simulink model "h175_model_cathode_harness_hctrl_basic"  (R2023a)
settings: Solver=VariableStepAuto  StartTime=0.0  StopTime=4750  RelTol=1e-2
InitFcn:
  | run("cathode_subsystem_parameters.m")
undefined symbols (not defined in the file or in its folder): sigbuilder_block
libraries: nesl_utility x12, fl_lib x10, simulink x5, slpidlib x2, eeGeneralControl x2, VariableTimeLowPassFilter x1
(part 2 of 2)

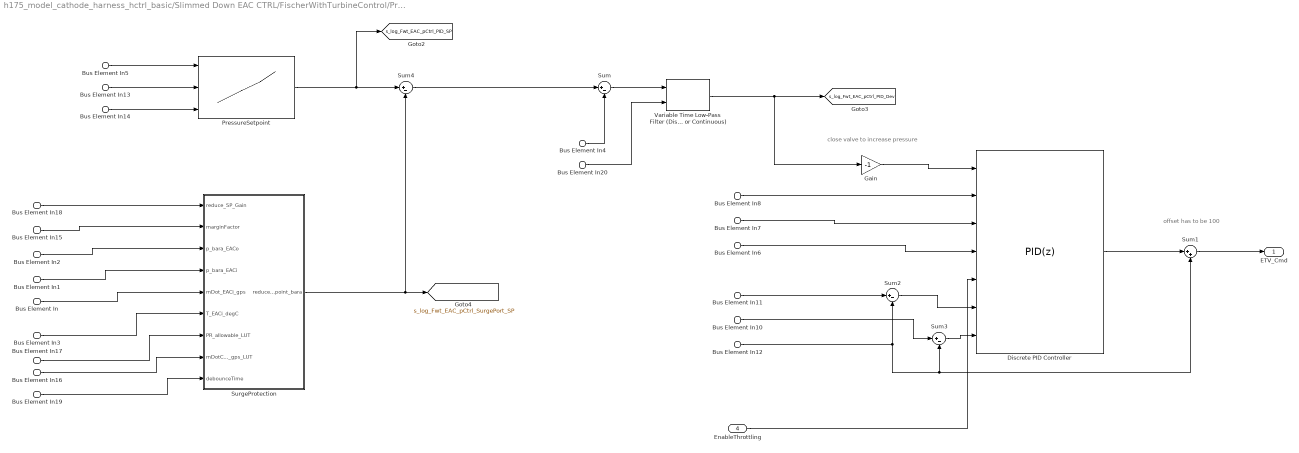
== system h175_model_cathode_harness_hctrl_basic/Slimmed Down EAC CTRL/FischerWithTurbineControl/PressureControl/AlternativeCathodePressureControl ==
  note: close valve to increase pressure
  note: offset has to be 100
  Bus Element In : Inport  PortName=CAT_Sensors  Element=b_mdotSens_EACi.s_mDot_gps_EACi_Get
  Bus Element In1 : Inport  PortName=CAT_Sensors  Element=b_pSens_EACi.s_p_bara_EACi_Get
  Bus Element In2 : Inport  PortName=CAT_Sensors  Element=b_pSens_EACo.s_p_bara_EACo_Get
  Bus Element In3 : Inport  PortName=CAT_Sensors  Element=b_TSens_EACi.s_T_degC_EACi_Get
  Bus Element In4 : Inport  PortName=CAT_Sensors  Element=b_pSens_CSti.s_p_bara_CSti_Get
  Bus Element In5 : Inport  Port=2  PortName=E_Sensors  Element=b_Sens_IVT.s_I_A_StN_Get
  Bus Element In6 : Inport  Port=3  PortName=EAC_Parameters  Element=p_Fwt_EAC_pCtrl_PID_D
  Bus Element In7 : Inport  Port=3  PortName=EAC_Parameters  Element=p_Fwt_EAC_pCtrl_PID_I
  Bus Element In8 : Inport  Port=3  PortName=EAC_Parameters  Element=p_Fwt_EAC_pCtrl_PID_P
  Bus Element In10 : Inport  Port=3  PortName=EAC_Parameters  Element=p_Fwt_EAC_pCtrl_PID_LowerLim_pos_per
  Bus Element In11 : Inport  Port=3  PortName=EAC_Parameters  Element=p_Fwt_EAC_pCtrl_PID_UpperLim_pos_per
  Bus Element In12 : Inport  Port=3  PortName=EAC_Parameters  Element=p_Fwt_EAC_pCtrl_PID_Offset_pos_per
  Bus Element In13 : Inport  Port=3  PortName=EAC_Parameters  Element=p_Fwt_EAC_pCtrl_SP_LUT_p_bara
  Bus Element In14 : Inport  Port=3  PortName=EAC_Parameters  Element=p_EAC_pCtrl_SP_LUT_I_A
  Bus Element In20 : Inport  Port=3  PortName=EAC_Parameters  Element=p_Fwt_EAC_pCtrl_PID_Filtr_T
  Bus Element In16 : Inport  Port=3  PortName=EAC_Parameters  Element=p_Fwt_EAC_pCtrl_SurgeProt_LUT_mDotCorr_gps
  Bus Element In17 : Inport  Port=3  PortName=EAC_Parameters  Element=p_Fwt_EAC_pCtrl_SurgeProt_LUT_PR
  Bus Element In15 : Inport  Port=3  PortName=EAC_Parameters  Element=p_Fwt_EAC_pCtrl_SurgeProt_PR_marginFactor
  Bus Element In18 : Inport  Port=3  PortName=EAC_Parameters  Element=p_Fwt_EAC_pCtrl_SurgeProt_redSP_Gain
  Bus Element In19 : Inport  Port=3  PortName=EAC_Parameters  Element=p_Fwt_EAC_pCtrl_SurgeProt_debounce_s
  EnableThrottling : Inport  Port=4
  Discrete PID Controller : slpidlib/PID Controller  Controller=PID  Form=Parallel  TimeDomain=Discrete-time  UseExternalTs=off  SampleTime=-1  IntegratorMethod=Trapezoidal  FilterMethod=Trapezoidal  ControllerParametersSource=external  P=1  I=1  UseKiTs=off  D=0  N=100  UseFilter=off  TunerSelectOption=Transfer Function Based (PID Tuner App)  InitialConditionSource=internal  InitialConditionForIntegrator=0  InitialConditionForFilter=0  DifferentiatorICPrevScaledInput=0  ExternalReset=either  TrackingMode=off  Kt=1  LimitOutput=on  SatLimitsSource=external  UpperSaturationLimit=inf  LowerSaturationLimit=-inf  LinearizeAsGain=off  AntiWindupMode=clamping  Kb=1  LimitIntegrator=off  UpperIntegratorSaturationLimit=inf  LowerIntegratorSaturationLimit=-inf  POutMin=[]  POutMax=[]  IOutMin=[]  IOutMax=[]  DOutMin=[]  DOutMax=[]  NOutMin=[]  NOutMax=[]  SumOutMin=[]  SumOutMax=[]  SaturationOutMin=[]  SaturationOutMax=[]  PParamMin=[]  PParamMax=[]  IParamMin=[]  IParamMax=[]  DParamMin=[]  DParamMax=[]  NParamMin=[]  NParamMax=[]  KbParamMin=[]  KbParamMax=[]  KtParamMin=[]  KtParamMax=[]  KbOutMin=[]  KbOutMax=[]  KtOutMin=[]  KtOutMax=[]  IntegratorOutMin=[]  IntegratorOutMax=[]  FilterOutMin=[]  FilterOutMax=[]  SumI1OutMin=[]  SumI1OutMax=[]  SumI2OutMin=[]  SumI2OutMax=[]  SumI3OutMin=[]  SumI3OutMax=[]  SumI4OutMin=[]  SumI4OutMax=[]  SumDOutMin=[]  SumDOutMax=[]  DifferentiatorOutMin=[]  DifferentiatorOutMax=[]  FilterDiffOutCoefMin=[]  FilterDiffOutCoefMax=[]  ReciprocalOutMin=[]  ReciprocalOutMax=[]  SumDenOutMin=[]  SumDenOutMax=[]  SumNumOutMin=[]  SumNumOutMax=[]  DivideOutMin=[]  DivideOutMax=[]  UdiffTsProdOutMin=[]  UdiffTsProdOutMax=[]  NTsProdOutMin=[]  NTsProdOutMax=[]  UintegralTsProdOutMin=[]  UintegralTsProdOutMax=[]  UngainTsProdOutMin=[]  UngainTsProdOutMax=[]  ClampingZeroOutDataTypeStr=Inherit: Inherit via back propagation  ClampingZeroOutMin=[]  ClampingZeroOutMax=[]  FilterDenConstantOutDataTypeStr=Inherit: Inherit via back propagation  FilterDenConstantOutMin=[]  FilterDenConstantOutMax=[]  PCopyOutDataTypeStr=Inherit: Inherit via back propagation  PCopyOutMin=[]  PCopyOutMax=[]  NCopyOutDataTypeStr=Inherit: Inherit via back propagation  NCopyOutMin=[]  NCopyOutMax=[]  IntegratorContinuousStateAttributes=''  IntegratorStateMustResolveToSignalObject=off  IntegratorRTWStateStorageClass=Auto  FilterContinuousStateAttributes=''  FilterStateMustResolveToSignalObject=off  FilterRTWStateStorageClass=Auto  ParallelPVariant=ExternalParameters  IdealPVariant=Disabled  IVariant=ExternalParameters  DVariant=ExternalParameters  IntegratorVariant=Discrete  SatVariant=External  AWVariant=DiscClampingParallel  PCopyVariant=Disabled  TRVariant=Disabled  FdbkBlocksVariant=Feedback  IdealPFdbkVariant=Passthrough  SatFdbkVariant=Passthrough  DerivativeFilterVariant=Differentiator  NVariant=Passthrough  NCopyVariant=Disabled_SignalSpec  FilterICVariant=InternalICsDifferentiator  IntegratorICVariant=InternalICs  ExternalResetVariant=ExternalReset  TRSumVariant=Passthrough  SumFdbkVariant=Enabled  SumVariant=Sum_PID  TsampFilterVariant=InternalTs  TsampNgainVariant=Passthrough  TsampIntegralVariant=Disabled_SignalSpec  ExternalSaturationOutDataTypeStr=Inherit: Same as second input
      settings: LibrarySourceBlock=simulink/Discrete/Discrete PID Controller
  Gain : Gain  Gain=-1
  PressureSetpoint : Lookup_n-D  NumberOfTableDimensions=1  BreakpointsForDimension1Source=Input port  BreakpointsForDimension1=[-5:5]  TableSource=Input port  Table=tanh([-5:5])  ExtrapMethod=Clip  InternalRulePriority=Speed  RndMeth=Simplest
      settings: InputPortMap=u0,p221,p5
  Sum{,2..4} (4 alike) : Sum  Inputs=|+-
  Sum1 : Sum  Inputs=|++
  SurgeProtection : Subsystem
  Variable Time Low-Pass Filter (Discrete or Continuous) : VariableTimeLowPassFilter/Variable Time Low-Pass Filter (Discrete or Continuous)  K=1  T=1  B=inf  A=-inf  init_option=Inherited from block input  x0=0  Ts=-1
      settings: LibrarySourceBlock=|
      | ee_sl_lib/General Control/Low-Pass Filter
      | (Discrete or Continuous)
  ETV_Cmd : Outport
  tag scope: s_log_Fwt_EAC_pCtrl_PID_Devi=global, s_log_Fwt_EAC_pCtrl_PID_SP=global, s_log_Fwt_EAC_pCtrl_SurgePort_SP=global
  wires:
  SurgeProtection/1(reducePressureSetpoint_bara) -> [s_log_Fwt_EAC_pCtrl_SurgePort_SP], Sum4/2
  Bus Element In19/1 -> SurgeProtection/9(debounceTime)
  Bus Element In16/1 -> SurgeProtection/8(mDotCorr_gps_LUT)
  Bus Element In17/1 -> SurgeProtection/7(PR_allowable_LUT)
  Bus Element In3/1 -> SurgeProtection/6(T_EACi_degC)
  Bus Element In/1 -> SurgeProtection/5(mDot_EACi_gps)
  Bus Element In1/1 -> SurgeProtection/4(p_bara_EACi)
  Bus Element In2/1 -> SurgeProtection/3(p_bara_EACo)
  Bus Element In15/1 -> SurgeProtection/2(marginFactor)
  Bus Element In18/1 -> SurgeProtection/1(reduce_SP_Gain)
  Bus Element In20/1 -> Variable Time Low-Pass Filter (Discrete or Continuous)/2
  Variable Time Low-Pass Filter (Discrete or Continuous)/1 -> [s_log_Fwt_EAC_pCtrl_PID_Devi], Gain/1
  Sum4/1 -> Sum/1
  PressureSetpoint/1 -> [s_log_Fwt_EAC_pCtrl_PID_SP], Sum4/1
  Bus Element In13/1 -> PressureSetpoint/2
  Bus Element In14/1 -> PressureSetpoint/3
  Discrete PID Controller/1 -> Sum1/1
  EnableThrottling/1 -> Discrete PID Controller/5
  Bus Element In7/1 -> Discrete PID Controller/3
  Sum/1 -> Variable Time Low-Pass Filter (Discrete or Continuous)/1
  Bus Element In8/1 -> Discrete PID Controller/2
  Sum3/1 -> Discrete PID Controller/7
  Bus Element In6/1 -> Discrete PID Controller/4
  Bus Element In11/1 -> Sum2/1
  Bus Element In12/1 -> Sum2/2, Sum3/2, Sum1/2
  Sum1/1 -> ETV_Cmd/1
  Sum2/1 -> Discrete PID Controller/6
  Bus Element In10/1 -> Sum3/1
  Gain/1 -> Discrete PID Controller/1
  Bus Element In5/1 -> PressureSetpoint/1
  Bus Element In4/1 -> Sum/2

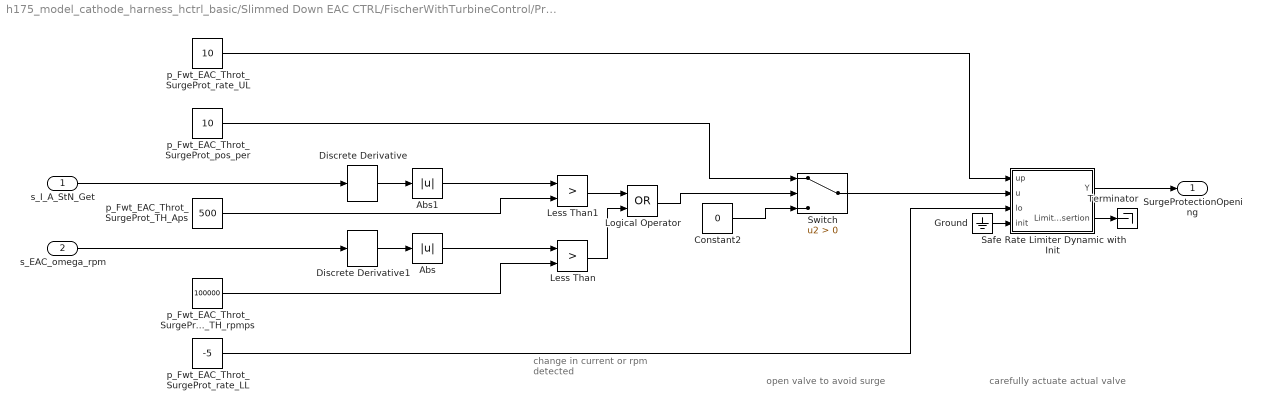
== system h175_model_cathode_harness_hctrl_basic/Slimmed Down EAC CTRL/FischerWithTurbineControl/PressureControl/SurgeProtection ==
  note: carefully actuate actual valve
  note: open valve to avoid surge
  note: change in current
      | or
      | rpm
      | detected
  s_I_A_StN_Get : Inport
  s_EAC_omega_rpm : Inport  Port=2
  Abs : Abs  SaturateOnIntegerOverflow=off
  Abs1 : Abs  SaturateOnIntegerOverflow=off
  Constant2 : Constant  Value=0  OutDataTypeStr=single
  Discrete Derivative : simulink/Discrete/Discrete Derivative  gainval=1.0  ICPrevScaledInput=0.0  OutMin=[]  OutMax=[]  OutDataType=fixdt(1, 16)  OutScaling=2^-10  DoSatur=off
  Discrete Derivative1 : simulink/Discrete/Discrete Derivative  gainval=1.0  ICPrevScaledInput=0.0  OutMin=[]  OutMax=[]  OutDataType=fixdt(1, 16)  OutScaling=2^-10  DoSatur=off
  Ground : Ground
  Less Than : RelationalOperator  Operator=>  OutDataTypeStr=boolean  RndMeth=Simplest  InputSameDT=off
  Less Than1 : RelationalOperator  Operator=>  OutDataTypeStr=boolean  RndMeth=Simplest  InputSameDT=off
  Logical Operator : Logic  Operator=OR  AllPortsSameDT=off  OutDataTypeStr=boolean
  Safe Rate Limiter Dynamic with Init : Subsystem  AncestorBlock=simulink/Discontinuities/Rate Limiter Dynamic  mask(Rate Limiter Dynamic){}
      mask help: Simulink:masks:RateLimiterDynamic_MD
  Switch : Switch  Criteria=u2 > Threshold  SaturateOnIntegerOverflow=off  InputSameDT=off
  Terminator : Terminator
  p_Fwt_EAC_Throt_SurgeProt_TH_Aps : Constant  Value=500
  p_Fwt_EAC_Throt_SurgeProt_TH_rpmps : Constant  Value=100000
  p_Fwt_EAC_Throt_SurgeProt_pos_per : Constant  Value=10
  p_Fwt_EAC_Throt_SurgeProt_rate_LL : Constant  Value=-5
  p_Fwt_EAC_Throt_SurgeProt_rate_UL : Constant  Value=10
  SurgeProtectionOpening : Outport
  wires:
  Abs1/1 -> Less Than1/1
  Discrete Derivative/1 -> Abs1/1
  p_Fwt_EAC_Throt_SurgeProt_TH_Aps/1 -> Less Than1/2
  s_I_A_StN_Get/1 -> Discrete Derivative/1
  Less Than1/1 -> Logical Operator/1
  Less Than/1 -> Logical Operator/2
  s_EAC_omega_rpm/1 -> Discrete Derivative1/1
  p_Fwt_EAC_Throt_SurgeProt_TH_rpmps/1 -> Less Than/2
  Switch/1 -> Safe Rate Limiter Dynamic with Init/2(u)
  Logical Operator/1 -> Switch/2
  Discrete Derivative1/1 -> Abs/1
  Constant2/1 -> Switch/3
  p_Fwt_EAC_Throt_SurgeProt_rate_LL/1 -> Safe Rate Limiter Dynamic with Init/3(lo)
  p_Fwt_EAC_Throt_SurgeProt_pos_per/1 -> Switch/1
  Abs/1 -> Less Than/1
  Safe Rate Limiter Dynamic with Init/1(Y) -> SurgeProtectionOpening/1
  p_Fwt_EAC_Throt_SurgeProt_rate_UL/1 -> Safe Rate Limiter Dynamic with Init/1(up)
  Ground/1 -> Safe Rate Limiter Dynamic with Init/4(init)
  Safe Rate Limiter Dynamic with Init/2(LimitsAssertion) -> Terminator/1

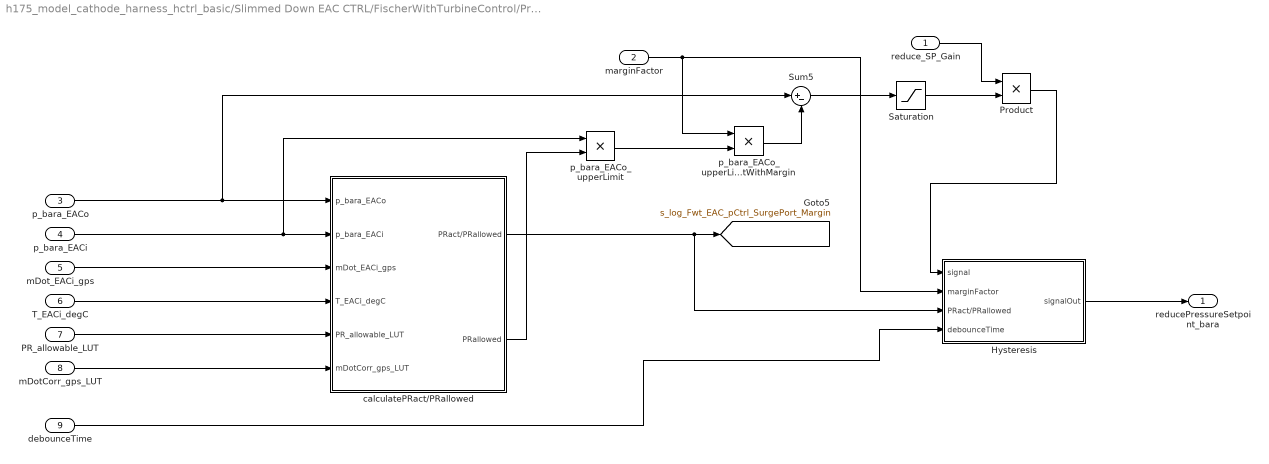
== system h175_model_cathode_harness_hctrl_basic/Slimmed Down EAC CTRL/FischerWithTurbineControl/PressureControl/AlternativeCathodePressureControl/SurgeProtection ==
  reduce_SP_Gain : Inport
  marginFactor : Inport  Port=2
  p_bara_EACo : Inport  Port=3
  p_bara_EACi : Inport  Port=4
  mDot_EACi_gps : Inport  Port=5
  T_EACi_degC : Inport  Port=6
  PR_allowable_LUT : Inport  Port=7
  mDotCorr_gps_LUT : Inport  Port=8
  debounceTime : Inport  Port=9
  Hysteresis : Subsystem
  Product : Product
  Saturation : Saturate  UpperLimit=inf  LowerLimit=0
  Sum5 : Sum  Inputs=|+-
  calculatePRact/PRallowed : Subsystem
  p_bara_EACo_upperLimit : Product
  p_bara_EACo_upperLimitWithMargin : Product
  reducePressureSetpoint_bara : Outport
  tag scope: s_log_Fwt_EAC_pCtrl_SurgePort_Margin=global
  wires:
  calculatePRact/PRallowed/2(PRallowed) -> p_bara_EACo_upperLimit/2
  calculatePRact/PRallowed/1(PRact/PRallowed) -> [s_log_Fwt_EAC_pCtrl_SurgePort_Margin], Hysteresis/3(PRact/PRallowed)
  mDotCorr_gps_LUT/1 -> calculatePRact/PRallowed/6(mDotCorr_gps_LUT)
  PR_allowable_LUT/1 -> calculatePRact/PRallowed/5(PR_allowable_LUT)
  T_EACi_degC/1 -> calculatePRact/PRallowed/4(T_EACi_degC)
  mDot_EACi_gps/1 -> calculatePRact/PRallowed/3(mDot_EACi_gps)
  Hysteresis/1(signalOut) -> reducePressureSetpoint_bara/1
  debounceTime/1 -> Hysteresis/4(debounceTime)
  Product/1 -> Hysteresis/1(signal)
  reduce_SP_Gain/1 -> Product/1
  p_bara_EACo_upperLimitWithMargin/1 -> Sum5/2
  Saturation/1 -> Product/2
  Sum5/1 -> Saturation/1
  p_bara_EACi/1 -> calculatePRact/PRallowed/2(p_bara_EACi), p_bara_EACo_upperLimit/1
  marginFactor/1 -> p_bara_EACo_upperLimitWithMargin/1, Hysteresis/2(marginFactor)
  p_bara_EACo/1 -> calculatePRact/PRallowed/1(p_bara_EACo), Sum5/1
  p_bara_EACo_upperLimit/1 -> p_bara_EACo_upperLimitWithMargin/2

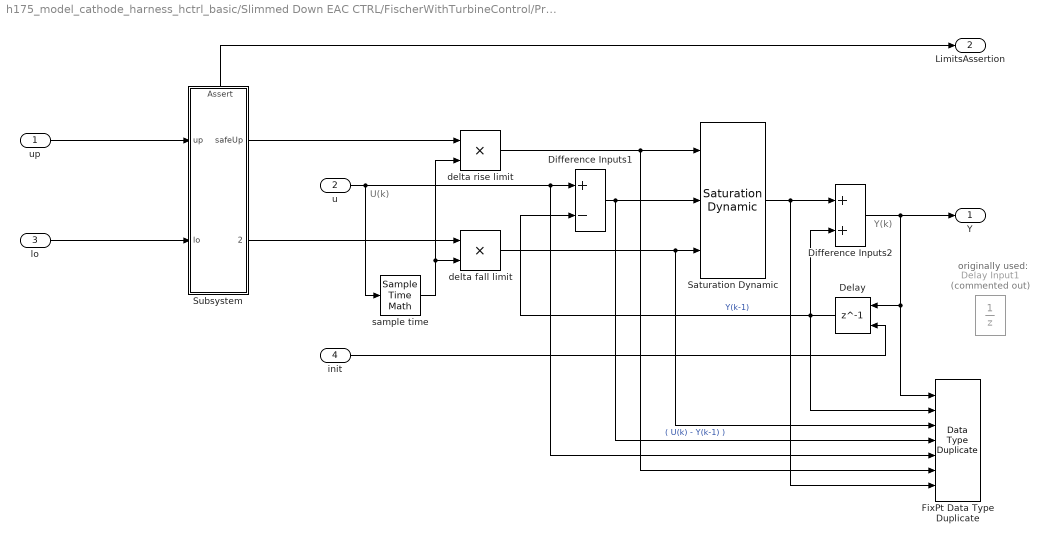
== system h175_model_cathode_harness_hctrl_basic/Slimmed Down EAC CTRL/FischerWithTurbineControl/PressureControl/SurgeProtection/Safe Rate Limiter Dynamic with Init ==
  note: Y(k)
  note: U(k)
  note: originally used:
  up : Inport
  u : Inport  Port=2
  lo : Inport  Port=3
  init : Inport  Port=4
  Delay : Delay  DelayLength=1  InitialConditionSource=Input port
      settings: InputPortMap=u0,p4
  Delay Input1 : UnitDelay  Description=Store in Global RAM  Commented=on  DisableCoverage=on  SampleTime=-1  HasFrameUpgradeWarning=on
  Difference Inputs1 : Sum  Description=Add in CPU  DisableCoverage=on  Inputs=+-  OutDataTypeStr=Inherit: Inherit via back propagation
  Difference Inputs2 : Sum  Description=Add in CPU  OutDataTypeStr=Inherit: Inherit via back propagation
  FixPt Data Type Duplicate : DataTypeDuplicate  DisableCoverage=on  NumInputPorts=7
  Saturation Dynamic : simulink/Discontinuities/Saturation Dynamic  OutMin=[]  OutMax=[]  OutDataTypeStr=Inherit: Same as second input  OutDataType=fixdt(1, 16)  OutScaling=2^-10  DoSatur=off
      settings: LibrarySourceBlock=|
      | simulink/Discontinuities/Rate Limiter
      | Dynamic/Saturation
      | Dynamic
  Subsystem : Subsystem
      settings: PortSchema="{\"entries\":[{\"content\":{\"sides\":[{\"content\":{\"connectorIds\":[\"In1\",\"In2\"]},\"type\":\"ConnectorPlacement.EquallySpacedRectSide\",\"uuid\":\"5f06f251-5ad3-4204-94b0-85cb08731d40\"},{\"content\":{\"connectorIds\":[\"Out1\",\"Out2\"],\"side\":\"RIGHT\"},\"type\":\"ConnectorPlacement.EquallySpacedRectSide\",\"uuid\":\"112376ac-3e5c-41b5-a3dd-1d4e75e1578c\"},{\"content\":{\"connectorIds\":[\"Out3\"],\"side\":\"TOP\"},\"type\":\"ConnectorPlacement.EquallySpacedRectSide\",\"uuid\":\"68a9a181-7018-40b9-8123-585370b895df\"}]},\"type\":\"ConnectorPlacement.EquallySpacedConnector\",\"uuid\":\"434bb119-8581-40d1-968f-b19607ab037e\"}],\"packageUris\":[\"http://schema.mathworks.com/mf0/Connector/R2020b\"],\"version\":\"1.0\"}"
  delta fall limit : Product  DisableCoverage=on  Inputs=**  OutDataTypeStr=Inherit: Inherit via back propagation  SaturateOnIntegerOverflow=on
  delta rise limit : Product  DisableCoverage=on  Inputs=**  OutDataTypeStr=Inherit: Inherit via back propagation  SaturateOnIntegerOverflow=on
  sample time : SampleTimeMath  DisableCoverage=on  TsampMathOp=Ts Only  weightValue=1
  Y : Outport  InitialOutput=0
  LimitsAssertion : Outport  Port=2
  wires:
  Subsystem/2(safeLow) -> delta fall limit/1
  Subsystem/1(safeUp) -> delta rise limit/1
  Subsystem/3(Assert) -> LimitsAssertion/1
  init/1 -> Delay/2
  Difference Inputs1/1 -> FixPt Data Type Duplicate/4, Saturation Dynamic/2  "( U(k) - Y(k-1) )"
  u/1 -> Difference Inputs1/1, FixPt Data Type Duplicate/5, sample time/1
  delta fall limit/1 -> FixPt Data Type Duplicate/3, Saturation Dynamic/3
  Saturation Dynamic/1 -> Difference Inputs2/1, FixPt Data Type Duplicate/7
  Delay/1 -> Difference Inputs2/2, Difference Inputs1/2, FixPt Data Type Duplicate/2  "Y(k-1)"
  Difference Inputs2/1 -> Y/1, Delay/1, FixPt Data Type Duplicate/1
  up/1 -> Subsystem/1(up)
  delta rise limit/1 -> FixPt Data Type Duplicate/6, Saturation Dynamic/1
  lo/1 -> Subsystem/2(lo)
  sample time/1 -> delta fall limit/2, delta rise limit/2

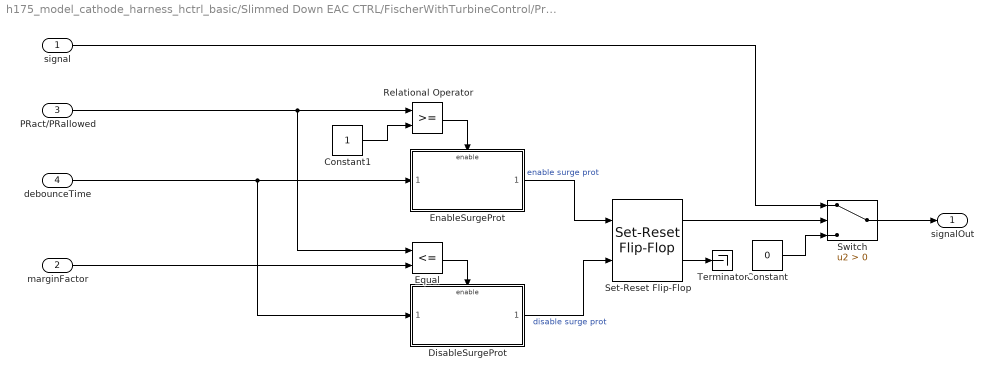
== system h175_model_cathode_harness_hctrl_basic/Slimmed Down EAC CTRL/FischerWithTurbineControl/PressureControl/AlternativeCathodePressureControl/SurgeProtection/Hysteresis ==
  signal : Inport
  marginFactor : Inport  Port=2
  PRact/PRallowed : Inport  Port=3
  debounceTime : Inport  Port=4
  Constant : Constant  Value=0  OutDataTypeStr=single
  Constant1 : Constant  OutDataTypeStr=single
  DisableSurgeProt : Subsystem  ReferencedSubsystem=EnabledTimer
  EnableSurgeProt : Subsystem  ReferencedSubsystem=EnabledTimer
  Equal : RelationalOperator  Operator=<=  OutDataTypeStr=boolean  RndMeth=Simplest  InputSameDT=off
  Relational Operator : RelationalOperator  OutDataTypeStr=boolean  RndMeth=Simplest  InputSameDT=off
  Set-Reset Flip-Flop : eeGeneralControl/Set-Reset Flip-Flop  LabelModeActiveChoice=Discrete  UndefState=Set  Q0=0  Ts=-1
      settings: LibrarySourceBlock=ee_sl_lib/General Control/Set-Reset Flip-Flop
  Switch : Switch  Criteria=u2 > Threshold  SaturateOnIntegerOverflow=off  InputSameDT=off
  Terminator : Terminator
  signalOut : Outport
  wires:
  marginFactor/1 -> Equal/2
  Switch/1 -> signalOut/1
  Relational Operator/1 -> EnableSurgeProt/Enable
  PRact/PRallowed/1 -> Relational Operator/1, Equal/1
  Constant/1 -> Switch/3
  signal/1 -> Switch/1
  DisableSurgeProt/1 -> Set-Reset Flip-Flop/2  "disable surge prot"
  Set-Reset Flip-Flop/1 -> Switch/2
  EnableSurgeProt/1 -> Set-Reset Flip-Flop/1  "enable surge prot"
  Set-Reset Flip-Flop/2 -> Terminator/1
  Constant1/1 -> Relational Operator/2
  debounceTime/1 -> EnableSurgeProt/1, DisableSurgeProt/1
  Equal/1 -> DisableSurgeProt/Enable

== system h175_model_cathode_harness_hctrl_basic/Slimmed Down EAC CTRL/FischerWithTurbineControl/PressureControl/AlternativeCathodePressureControl/SurgeProtection/calculatePRact//PRallowed ==
  p_bara_EACo : Inport
  p_bara_EACi : Inport  Port=2
  mDot_EACi_gps : Inport  Port=3
  T_EACi_degC : Inport  Port=4
  PR_allowable_LUT : Inport  Port=5
  mDotCorr_gps_LUT : Inport  Port=6
  Divide : Product  Inputs=*/
  PressureRatioActual : Product  Inputs=*/
  PressureRatioAllowable : Lookup_n-D  NumberOfTableDimensions=1  BreakpointsForDimension1Source=Input port  BreakpointsForDimension1=[-5:5]  TableSource=Input port  Table=tanh([-5:5])  ExtrapMethod=Clip  InternalRulePriority=Speed  RndMeth=Simplest
      settings: InputPortMap=u0,p221,p5
  bara --> kPa : Gain  Gain=100
  bara --> kPa1 : Gain  Gain=100
  calculateCorrectedMassflow : MATLAB Function  TreatAsAtomicUnit=on
  PRact/PRallowed : Outport
  PRallowed : Outport  Port=2
  wires:
  p_bara_EACo/1 -> bara --> kPa1/1
  p_bara_EACi/1 -> bara --> kPa/1
  Divide/1 -> PRact/PRallowed/1
  mDotCorr_gps_LUT/1 -> PressureRatioAllowable/3
  PR_allowable_LUT/1 -> PressureRatioAllowable/2
  T_EACi_degC/1 -> calculateCorrectedMassflow/2(T_EACi_degC)
  mDot_EACi_gps/1 -> calculateCorrectedMassflow/1(mDot_EACi_gps)
  bara --> kPa1/1 -> PressureRatioActual/1
  calculateCorrectedMassflow/1(mDot_corr_EACi_gps) -> PressureRatioAllowable/1
  PressureRatioActual/1 -> Divide/1
  PressureRatioAllowable/1 -> PRallowed/1, Divide/2
  bara --> kPa/1 -> calculateCorrectedMassflow/3(p_EACi_kPa), PressureRatioActual/2

== system h175_model_cathode_harness_hctrl_basic/Slimmed Down EAC CTRL/FischerWithTurbineControl/PressureControl/SurgeProtection/Safe Rate Limiter Dynamic with Init/Subsystem ==
  up : Inport
  lo : Inport  Port=2
  Check Static Lower Bound : simulink/Model Verification/Check Static  Lower Bound  Description=0 <= u  min=0  min_included=on  enabled=on  stopWhenAssertionFail=off  export=on  icon=graphic
  Check Static Upper Bound : simulink/Model Verification/Check Static  Upper Bound  Description=u <= 0  max=0  max_included=on  enabled=on  stopWhenAssertionFail=off  export=on  icon=graphic
  Gain1 : Gain  Gain=-1
  Gain2 : Gain  Gain=-1
  Logical Operator : Logic  AllPortsSameDT=off  OutDataTypeStr=boolean
  Switch : Switch  Criteria=u2 > Threshold  SaturateOnIntegerOverflow=off  InputSameDT=off
  Switch1 : Switch  Criteria=u2 > Threshold  SaturateOnIntegerOverflow=off  InputSameDT=off
  safeUp : Outport
  safeLow : Outport  Port=2
  Assert : Outport  Port=3
  wires:
  Gain1/1 -> Switch/3
  Gain2/1 -> Switch1/3
  Switch/1 -> safeUp/1
  lo/1 -> Check Static Upper Bound/1, Gain2/1, Switch1/1
  up/1 -> Check Static Lower Bound/1, Gain1/1, Switch/1
  Logical Operator/1 -> Assert/1
  Switch1/1 -> safeLow/1
  Check Static Lower Bound/1 -> Logical Operator/1, Switch/2
  Check Static Upper Bound/1 -> Switch1/2, Logical Operator/2

== matlab function h175_model_cathode_harness_hctrl_basic/Plant_Sensors/EAC_Theo_Power/MATLAB Function ==
  data: u input; y output; data input
function y = fcn(u, data)

y = (u^data)-1;

== matlab function h175_model_cathode_harness_hctrl_basic/Plant_Sensors/EAT_Theo_Power/MATLAB Function ==
  data: u input; y output; data input
function y = fcn(u, data)

y = (u^data)-1;

== matlab function h175_model_cathode_harness_hctrl_basic/Slimmed Down EAC CTRL/Subsystem/calculation_theoretical_massflow/theoretical_massflow ==
  data: n_cells input; s_mDot_0_gps output; M_O2 input; F input; x_m_O2 input; I_SFC input
function s_mDot_0_gps = calculation_theoretical_massflow(n_cells, M_O2, F, x_m_O2, I_SFC)

    s_mDot_0_gps = I_SFC * ((n_cells * M_O2)/(4*F * (x_m_O2/100)));

end %function

== stateflow chart h175_model_cathode_harness_hctrl_basic/Slimmed Down EAC CTRL/TurbineDrainSequencing/TurbineDrainScheduler ==
  state Timer [parallel]
    settings: executionOrder=1
    state init
      %dummy state to waist one time step
      en:
      trigger = 0;
    state closed
      en:
      trigger = 0;
    state opened
      en:
      trigger = 1;
    (default) -> init
    init -> Timer.closed : [trigger==0]
    Timer.closed -> Timer.opened : after(period,sec)
    Timer.opened -> Timer.closed : [trigger==1]
  state Opener [parallel]
    settings: executionOrder=2
    state closed
      en:
      valveCommand = DVLV_STATE.Closed;
    state opened
      en:
      valveCommand = DVLV_STATE.Open;
    (default) -> Opener.closed
    Opener.closed -> Opener.opened : [trigger==1 && ...
        | openTime > 0]
    Opener.opened -> Opener.closed : after(openTime,sec)
  data: period input; openTime input; valveCommand output Enum: DVLV_STATE; trigger local

== matlab function h175_model_cathode_harness_hctrl_basic/Slimmed Down EAC CTRL/FischerWithTurbineControl/PressureControl/AlternativeCathodePressureControl/SurgeProtection/calculatePRact//PRallowed/calculateCorrectedMassflow ==
  data: mDot_EACi_gps input; mDot_corr_EACi_gps output; T_EACi_degC input; p_EACi_kPa input
function mDot_corr_EACi_gps = fcn(mDot_EACi_gps, T_EACi_degC, p_EACi_kPa)

mDot_corr_EACi_gps = mDot_EACi_gps * sqrt( (273.15 + T_EACi_degC) / 298 ) / ( p_EACi_kPa / 101.325 ) ;
